simulink model "Ctrl_For_HRV_20260625"  (R2024b)
settings: Solver=ode4  StartTime=0.0  StopTime=28  FixedStep=0.02  RelTol=1e-3
InitFcn:
  | Parameter;
values from neighbouring files (symbols this model uses):
  h_alpha = h_1    (= 0.02)    [Parameter.m]
  h_beta = h_1    (= 0.02)    [Parameter.m]
  h_miu = h_1    (= 0.02)    [Parameter.m]
  h_p = h_1    (= 0.02)    [Parameter.m]
  h_q = h_1    (= 0.02)    [Parameter.m]
  h_r = h_1    (= 0.02)    [Parameter.m]
  r_alpha = r_1    (= 0.04)    [Parameter.m]
  r_beta = r_1    (= 0.04)    [Parameter.m]
  r_miu = r_3    (= 0.03)    [Parameter.m]
  r_p = r_2    (= 1.28)    [Parameter.m]
  r_q = r_2    (= 1.28)    [Parameter.m]
  r_r = r_2    (= 1.28)    [Parameter.m]
  xishu = 0    [Parameter.m]
  xishu_D_0 = 0.3    [Parameter.m]
  xishu_L_0 = 0.2    [Parameter.m]
  xishu_l_0 = 0.23    [Parameter.m]
  xishu_m_0 = 0.17    [Parameter.m]
  xishu_n_0 = 0.09    [Parameter.m]
  xishu_Y_0 = 0.14    [Parameter.m]
undefined symbols (not defined in the file or in its folder): CCI_DUI_AngleRate_Controller, CCI_DUI_FlowAngle_Controller, fhan, PNG_2026_6_23
libraries: simulink x12
(part 2 of 2)

== matlab function Ctrl_For_HRV_20260625/MATLAB Function2 ==
  data: ny output; nz output; position_t input; vt input; hgv_states input; theta_f input; kai_f input
function [ny, nz] = Prop_guidance(position_t, vt, hgv_states, theta_f, kai_f)            
                                                                                        % Proportional navigation in HRV_Model coordinates: X forward, Y lateral, H vertical.    
                                                                                            H = hgv_states(1); lat = hgv_states(3); V = max(hgv_states(4), 1.0);                 
                                                                                            theta = hgv_states(5); psi = hgv_states(6);                                          
                                                                                            X = hgv_states(7); alt = hgv_states(8); Y = hgv_states(9);                           
                                                                                            rx = position_t(1) - X; ry = position_t(2) - Y; rh = position_t(3) - alt;            
                                                                                            vx = V*cos(theta)*cos(psi); vy = V*cos(theta)*sin(psi); vh = V*sin(theta);           
                                                                                            vrx = vt(1) - vx; vry = vt(2) - vy; vrh = vt(3) - vh;                                
                                                                                            earth_r = 6371000; omega = 7.292116e-5; Rearth = earth_r + H; g = gravityLocal(H);   
                                                                                            r2 = max(rx^2 + ry^2 + rh^2, 1.0); r = sqrt(r2);                                     
                                                                                            rhoriz2 = max(rx^2 + ry^2, 1.0);                                                     
                                                                                            closingRaw = -(rx*vrx + ry*vry + rh*vrh)/r;                                          
                                                                                            closing = max(closingRaw, 50.0);                                                     
                                                                                            tgo = min(max(r/closing, 1.5), 120.0);                                               
                                                                                            rangeXH2 = max(rx^2 + rh^2, 1.0);                                                    
                                                                                            qTheta = atan2(rh, rx); qPsi = atan2(ry, rx);                                        
                                                                                            qThetaDot = (rx*vrh - rh*vrx)/rangeXH2;                                              
                                                                                            qPsiDot = (rx*vry - ry*vrx)/rhoriz2;                                                 
                                                                                            thetaErr = wrapToPiLocal(qTheta - theta); psiErr = wrapToPiLocal(qPsi - psi);        
                                                                                            Ntheta = 3.2; Npsi = 2.2; Ktheta = 0.9; Kpsi = 0.35;                                 
                                                                                            aTheta = Ntheta*closing*qThetaDot + Ktheta*V*thetaErr/tgo;                           
                                                                                            aPsi = Npsi*closing*qPsiDot + Kpsi*V*cos(theta)*psiErr/tgo;                          
                                                                                            aTheta = saturate(aTheta, -4.8*g, 0.30*g);                                           
                                                                                            aPsi = saturate(aPsi, -0.18*g, 0.18*g);                                              
                                                                                            terminalScale = terminalFade(r, closingRaw);                                         
                                                                                            aTheta = terminalScale*aTheta;                                                       
                                                                                            aPsi = terminalScale*aPsi;                                                           
                                                                                            geomTheta = V*cos(theta)/Rearth + 2*omega*cos(lat)*sin(psi) ...                      
                                                                                                + omega^2*Rearth*cos(lat)*(cos(theta)*cos(lat) + sin(theta)*cos(psi)*sin(lat))/V;
                                                                                            geomPsi = V*cos(theta)*sin(psi)*tan(lat)/Rearth ...                                  
                                                                                                + 2*omega*(sin(lat) - cos(lat)*cos(psi)*tan(theta)) ...                          
                                                                                                + omega^2*Rearth*cos(lat)*sin(lat)*sin(psi)/(V*cos(theta));                      
                                                                                            ny = aTheta/g + cos(theta) - (V/g)*geomTheta;                                        
                                                                                            nz = aPsi/g - (V*cos(theta)/g)*geomPsi;                                              
                                                                                            ny = saturate(ny, -4.30, 1.25);                                                      
                                                                                            nz = saturate(nz, -0.18, 0.18);                                                      
                                                                                            dummy = theta_f + kai_f; %#ok<NASGU>                                                 
                                                                                        end                                                                                      
                                                                                        function scale = terminalFade(r, closingRaw)                                             
                                                                                            fadeStart = 180.0; fadeEnd = 30.0;                                                   
                                                                                            if closingRaw <= 0.0                                                                 
                                                                                                scale = 0.0;                                                                     
                                                                                            else                                                                                 
                                                                                                x = saturate((r - fadeEnd)/(fadeStart - fadeEnd), 0.0, 1.0);                     
                                                                                                scale = x*x*(3.0 - 2.0*x);                                                       
                                                                                            end                                                                                  
                                                                                        end                                                                                      
                                                                                        function y = saturate(x, lo, hi)                                                         
                                                                                            y = min(max(x, lo), hi);                                                             
                                                                                        end                                                                                      
                                                                                        function ang = wrapToPiLocal(ang)                                                        
                                                                                            ang = mod(ang + pi, 2*pi) - pi;                                                      
                                                                                        end                                                                                      
                                                                                        function g = gravityLocal(H)                                                             
                                                                                            earth_r = 6371000; g0 = 9.806; g = (earth_r/(earth_r + H))^2*g0;                     
                                                                                        end
